simulink library "ude"  (Simulink 8.2)
settings: Solver=ode1  StartTime=0.0  StopTime=Inf  FixedStep=0.001  RelTol=1e-3
PostLoadFcn:
  | , if any(exist('dsrtsu_mdlpostloadfcn', 'file') == [2, 3, 6]), try dsrtsu_mdlpostloadfcn('Execute', bdroot); catch fprintf('Error in PostLoadFcn (dsrtsu_mdlpostloadfcn) for model "%s":\n %s\n', bdroot, lasterr); end, end,
undefined symbols (not defined in the file or in its folder): FALSE, TRUE
libraries: hcu_lib x4, simulink x2
(part 2 of 2)

== system ude/UDE/ude/Procr_RadarSignals/Procr_RadarSignals/obj 7 ID compare ==
  ADAS_CAN_Rx : Inport
  Bus Selector1 : BusSelector  OutputSignals=SENP58.RadarTar7_ID_A,SENP59.RadarTar7_ID_B
  Constant : Constant  Value=0
  Relational Operator : RelationalOperator  Operator===  OutDataTypeStr=boolean
  Switch : Switch  Criteria=u2 ~= 0
  VHAL_RadarObj7ID_enum : Outport
  wires:
  Constant/1 -> Switch/3
  Relational Operator/1 -> Switch/2
  Switch/1 -> VHAL_RadarObj7ID_enum/1
  ADAS_CAN_Rx/1 -> Bus Selector1/1
  Bus Selector1/1 -> Relational Operator/1, Switch/1  "<RadarTar7_ID_A>"
  Bus Selector1/2 -> Relational Operator/2  "<RadarTar7_ID_B>"

== system ude/UDE/ude/Procr_RadarSignals/Procr_RadarSignals/obj 7 Status test ==
  ADAS_CAN_Rx : Inport
  Bus Selector1 : BusSelector  OutputSignals=SENP59.RadarTar7_DynProp
  Invalid : Constant  Value=0
  Multiport Switch : MultiPortSwitch  DataPortOrder=Zero-based contiguous  Inputs=4
  moving : Constant  Value=3
  stopped : Constant  Value=2
  unclassified : Constant  Value=0
  VHAL_RadarObj7Status_enum : Outport
  wires:
  Multiport Switch/1 -> VHAL_RadarObj7Status_enum/1
  Invalid/1 -> Multiport Switch/5
  moving/1 -> Multiport Switch/4
  stopped/1 -> Multiport Switch/3
  unclassified/1 -> Multiport Switch/2
  Bus Selector1/1 -> Multiport Switch/1  "<RadarTar7_DynProp>"
  ADAS_CAN_Rx/1 -> Bus Selector1/1

== system ude/UDE/ude/Procr_RadarSignals/Procr_RadarSignals/obj 7 valid test ==
  ADAS_CAN_Rx : Inport
  Bus Selector1 : BusSelector  OutputSignals=SENP59.RadarTar7_MeasStat
  Constant : Constant  Value=FALSE
  Constant1 : Constant  Value=TRUE
  Constant3 : Constant  Value=FALSE
  Constant4 : Constant  Value=TRUE
  Multiport Switch : MultiPortSwitch  DataPortOrder=Zero-based contiguous  Inputs=4
  VHAL_RadarObj7Valid_flg : Outport
  wires:
  Multiport Switch/1 -> VHAL_RadarObj7Valid_flg/1
  Constant3/1 -> Multiport Switch/5
  Constant4/1 -> Multiport Switch/4
  Constant1/1 -> Multiport Switch/3
  Constant/1 -> Multiport Switch/2
  Bus Selector1/1 -> Multiport Switch/1  "<RadarTar7_MeasStat>"
  ADAS_CAN_Rx/1 -> Bus Selector1/1

== system ude/UDE/ude/Procr_RadarSignals/Procr_RadarSignals/obj 7 width test ==
  VHAL_RadarObj7Valid_flg : Inport
  Constant : Constant  Value=0
  Constant1 : Constant  Value=2
  Multiport Switch : MultiPortSwitch  DataPortOrder=Zero-based contiguous  Inputs=2
  VHAL_RadarObj7Width_m : Outport
  wires:
  Multiport Switch/1 -> VHAL_RadarObj7Width_m/1
  Constant1/1 -> Multiport Switch/3
  Constant/1 -> Multiport Switch/2
  VHAL_RadarObj7Valid_flg/1 -> Multiport Switch/1

== system ude/UDE/ude/Procr_RadarSignals/Procr_RadarSignals/obj 8 ID compare ==
  ADAS_CAN_Rx : Inport
  Bus Selector1 : BusSelector  OutputSignals=SENP60.RadarTar8_ID_A,SENP61.RadarTar8_ID_B
  Constant : Constant  Value=0
  Relational Operator : RelationalOperator  Operator===  OutDataTypeStr=boolean
  Switch : Switch  Criteria=u2 ~= 0
  VHAL_RadarObj8ID_enum : Outport
  wires:
  Bus Selector1/2 -> Relational Operator/2  "<RadarTar8_ID_B>"
  Bus Selector1/1 -> Switch/1, Relational Operator/1  "<RadarTar8_ID_A>"
  ADAS_CAN_Rx/1 -> Bus Selector1/1
  Switch/1 -> VHAL_RadarObj8ID_enum/1
  Relational Operator/1 -> Switch/2
  Constant/1 -> Switch/3

== system ude/UDE/ude/Procr_RadarSignals/Procr_RadarSignals/obj 8 Status test ==
  ADAS_CAN_Rx : Inport
  Bus Selector1 : BusSelector  OutputSignals=SENP61.RadarTar8_DynProp
  Invalid : Constant  Value=0
  Multiport Switch : MultiPortSwitch  DataPortOrder=Zero-based contiguous  Inputs=4
  moving : Constant  Value=3
  stopped : Constant  Value=2
  unclassified : Constant  Value=0
  VHAL_RadarObj8Status_enum : Outport
  wires:
  ADAS_CAN_Rx/1 -> Bus Selector1/1
  Bus Selector1/1 -> Multiport Switch/1  "<RadarTar8_DynProp>"
  unclassified/1 -> Multiport Switch/2
  stopped/1 -> Multiport Switch/3
  moving/1 -> Multiport Switch/4
  Invalid/1 -> Multiport Switch/5
  Multiport Switch/1 -> VHAL_RadarObj8Status_enum/1

== system ude/UDE/ude/Procr_RadarSignals/Procr_RadarSignals/obj 8 valid test ==
  ADAS_CAN_Rx : Inport
  Bus Selector1 : BusSelector  OutputSignals=SENP61.RadarTar8_MeasStat
  Constant : Constant  Value=FALSE
  Constant1 : Constant  Value=TRUE
  Constant3 : Constant  Value=FALSE
  Constant4 : Constant  Value=TRUE
  Multiport Switch : MultiPortSwitch  DataPortOrder=Zero-based contiguous  Inputs=4
  VHAL_RadarObj8Valid_flg : Outport
  wires:
  ADAS_CAN_Rx/1 -> Bus Selector1/1
  Bus Selector1/1 -> Multiport Switch/1  "<RadarTar8_MeasStat>"
  Constant/1 -> Multiport Switch/2
  Constant1/1 -> Multiport Switch/3
  Constant4/1 -> Multiport Switch/4
  Constant3/1 -> Multiport Switch/5
  Multiport Switch/1 -> VHAL_RadarObj8Valid_flg/1

== system ude/UDE/ude/Procr_RadarSignals/Procr_RadarSignals/obj 8 width test ==
  VHAL_RadarObj8Valid_flg : Inport
  Constant : Constant  Value=0
  Constant1 : Constant  Value=2
  Multiport Switch : MultiPortSwitch  DataPortOrder=Zero-based contiguous  Inputs=2
  VHAL_RadarObj8Width_m : Outport
  wires:
  VHAL_RadarObj8Valid_flg/1 -> Multiport Switch/1
  Constant/1 -> Multiport Switch/2
  Constant1/1 -> Multiport Switch/3
  Multiport Switch/1 -> VHAL_RadarObj8Width_m/1
